simulink model "BCD_to7"  (R2021b)
settings: Solver=VariableStepAuto  StartTime=0.0  StopTime=10.0  RelTol=1e-3
values from neighbouring files (symbols this model uses):
  W = str2double(num_bin(1))    [HDTask2.m]
  X = str2double(num_bin(2))    [HDTask2.m]    (also in PBTask5p1.m = or(not(and1), and2); PBTask5p2.m = and(not(or(A, B)), C))
  Y = str2double(num_bin(3))    [HDTask2.m]    (also in PBTask5p2.m = or(and(and(A, not(B)), C), and(not(A), D), and(C, not(D))))
  Z = str2double(num_bin(4))    [HDTask2.m]
settings Model: Creator=ut-kr  LastModifiedBy=ut-kr

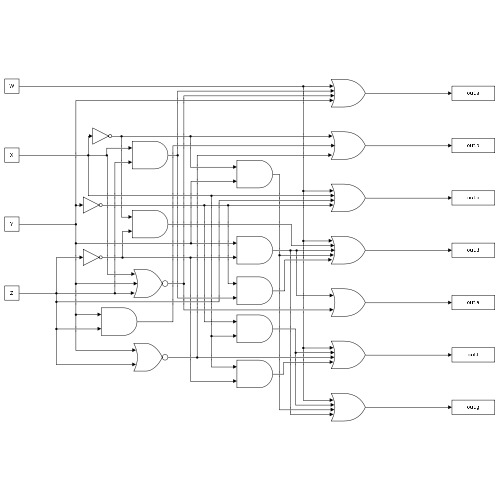
[thumbnail: Simulink's stored preview of the top-level diagram]
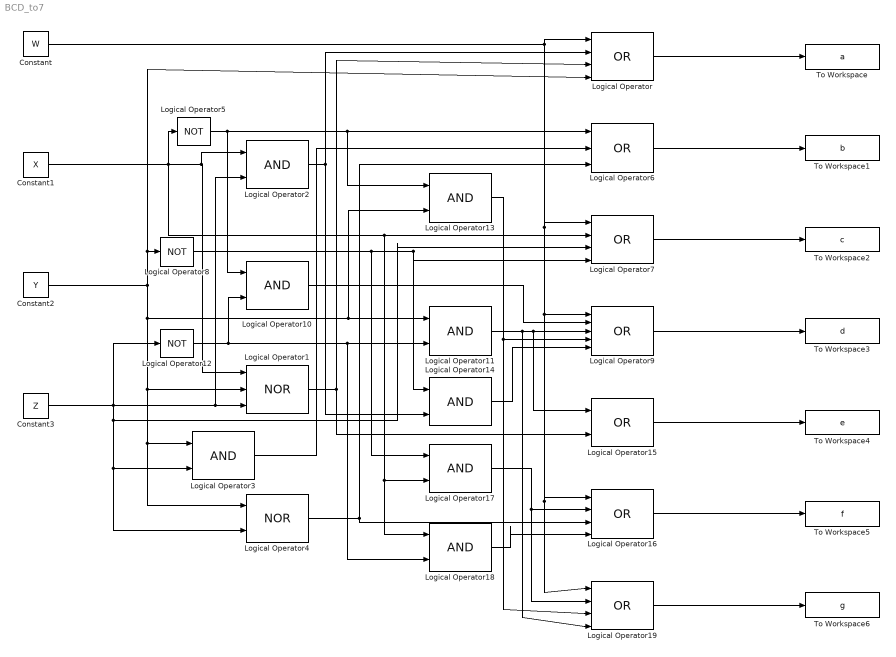
== system BCD_to7 ==
  Constant : Constant  Value=W
  Constant1 : Constant  Value=X
  Constant2 : Constant  Value=Y
  Constant3 : Constant  Value=Z
  Logical Operator{,7,16,19} (4 alike) : Logic  Operator=OR  Inputs=4  IconShape=distinctive  AllPortsSameDT=off  OutDataTypeStr=boolean
  Logical Operator1 : Logic  Operator=NOR  Inputs=3  IconShape=distinctive  AllPortsSameDT=off  OutDataTypeStr=boolean
  Logical Operator{2..3,10..11,13..14,17..18} (8 alike) : Logic  IconShape=distinctive  AllPortsSameDT=off  OutDataTypeStr=boolean
  Logical Operator12 : Logic  Operator=NOT  Inputs=3  IconShape=distinctive  AllPortsSameDT=off  OutDataTypeStr=boolean
  Logical Operator15 : Logic  Operator=OR  IconShape=distinctive  AllPortsSameDT=off  OutDataTypeStr=boolean
  Logical Operator4 : Logic  Operator=NOR  IconShape=distinctive  AllPortsSameDT=off  OutDataTypeStr=boolean
  Logical Operator5 : Logic  Operator=NOT  Inputs=3  IconShape=distinctive  AllPortsSameDT=off  OutDataTypeStr=boolean
  Logical Operator6 : Logic  Operator=OR  Inputs=3  IconShape=distinctive  AllPortsSameDT=off  OutDataTypeStr=boolean
  Logical Operator8 : Logic  Operator=NOT  Inputs=3  IconShape=distinctive  AllPortsSameDT=off  OutDataTypeStr=boolean
  Logical Operator9 : Logic  Operator=OR  Inputs=5  IconShape=distinctive  AllPortsSameDT=off  OutDataTypeStr=boolean
  To Workspace : ToWorkspace  VariableName=a  SaveFormat=Timeseries  SampleTime=-1
  To Workspace1 : ToWorkspace  VariableName=b  SaveFormat=Timeseries  SampleTime=-1
  To Workspace2 : ToWorkspace  VariableName=c  SaveFormat=Timeseries  SampleTime=-1
  To Workspace3 : ToWorkspace  VariableName=d  SaveFormat=Timeseries  SampleTime=-1
  To Workspace4 : ToWorkspace  VariableName=e  SaveFormat=Timeseries  SampleTime=-1
  To Workspace5 : ToWorkspace  VariableName=f  SaveFormat=Timeseries  SampleTime=-1
  To Workspace6 : ToWorkspace  VariableName=g  SaveFormat=Timeseries  SampleTime=-1
  wires:
  Constant/1 -> Logical Operator19/1, Logical Operator16/1, Logical Operator9/1, Logical Operator7/1, Logical Operator/1
  Constant1/1 -> Logical Operator18/1, Logical Operator17/2, Logical Operator7/2, Logical Operator5/1, Logical Operator2/1, Logical Operator1/1
  Constant2/1 -> Logical Operator/4, Logical Operator8/1, Logical Operator11/1, Logical Operator13/2, Logical Operator4/1, Logical Operator3/1, Logical Operator1/2
  Constant3/1 -> Logical Operator4/2, Logical Operator3/2, Logical Operator7/3, Logical Operator12/1, Logical Operator1/3, Logical Operator2/2
  Logical Operator2/1 -> Logical Operator14/2, Logical Operator/2
  Logical Operator1/1 -> Logical Operator/3, Logical Operator15/2
  Logical Operator/1 -> To Workspace/1
  Logical Operator5/1 -> Logical Operator6/1, Logical Operator13/1, Logical Operator10/1
  Logical Operator3/1 -> Logical Operator6/2
  Logical Operator4/1 -> Logical Operator16/3, Logical Operator6/3
  Logical Operator6/1 -> To Workspace1/1
  Logical Operator8/1 -> Logical Operator17/1, Logical Operator7/4, Logical Operator14/1
  Logical Operator7/1 -> To Workspace2/1
  Logical Operator11/1 -> Logical Operator19/4, Logical Operator15/1, Logical Operator9/3
  Logical Operator12/1 -> Logical Operator10/2, Logical Operator18/2, Logical Operator11/2
  Logical Operator13/1 -> Logical Operator9/4, Logical Operator19/3
  Logical Operator14/1 -> Logical Operator9/5
  Logical Operator17/1 -> Logical Operator19/2, Logical Operator16/2
  Logical Operator18/1 -> Logical Operator16/4
  Logical Operator19/1 -> To Workspace6/1
  Logical Operator16/1 -> To Workspace5/1
  Logical Operator15/1 -> To Workspace4/1
  Logical Operator9/1 -> To Workspace3/1
  Logical Operator10/1 -> Logical Operator9/2
